simulink model "COMH_Test"  (R2016b)
settings: Solver=VariableStepAuto  StartTime=0.0  StopTime=55  RelTol=1e-3  EnableMultiTasking=on
undefined symbols (not defined in the file or in its folder): CAL_EncoderSampleTime, CAL_fullCircle_DEG, CAL_MeasureNoise, CAL_ProcessNoise, CAL_ROB_ERRVAL, CAL_ROBO_LENG_mm, CAL_thetaGain, COMH, Compass_Handler, CONST_EnableDelay, CONST_ZERO_UINT16, CONST_ZeroDeg, ENU_ROB_NONE, sigbuilder_block
libraries: simulink_need_slupdate x1, ThetaOverFlowFilter x1, movingAverage_1ms_to_5ms x1, simulink x1
settings Model: Creator=oelkawok  LastModifiedBy=oelkawok
settings OptimizationCC: LifeSpan=inf
settings DebuggingCC: SFUnexpectedBacktrackingDiag=warning  SFNoUnconditionalDefaultTransitionDiag=warning  SFExecutionAtInitializationDiag=none
settings GRTTargetCC: TargetLangStandard=C89/C90 (ANSI)  GeneratePreprocessorConditionals=Disable all
settings ConfigComp: CovMetricSettings=dw  CovHtmlReporting=on  CovSaveCumulativeToWorkspaceVar=on  CovSaveSingleToWorkspaceVar=on  CovExternalEMLEnable=off

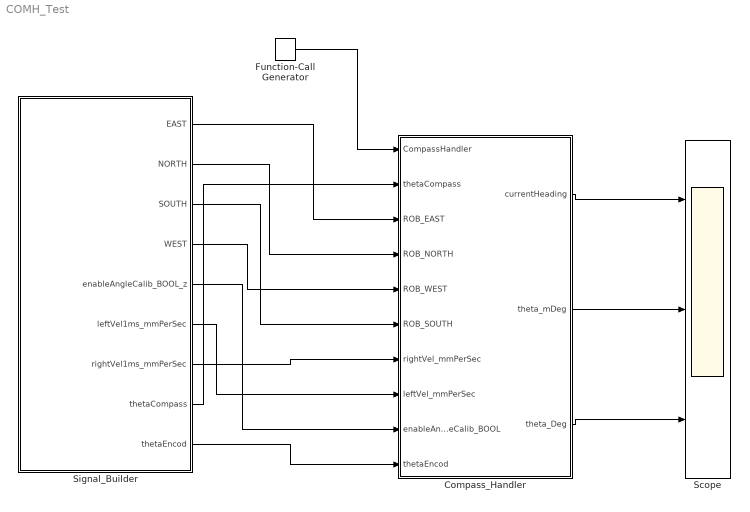
== system COMH_Test ==
  Compass_Handler : Subsystem  AncestorBlock=COMH/Compass_Handler
  Function-Call Generator : simulink/Ports & Subsystems/Function-Call Generator  sample_time=0.005  numberOfIterations=1
  Scope : Scope  NumInputPorts=3
  Signal_Builder : Subsystem  Tag=STV Subsys  LoadFcn=sigbuilder_block('load',[5.4 30 1141.2 522.6 ]);  StartFcn=sigbuilder_block('start');  StopFcn=sigbuilder_block('stop');  ClipboardFcn=sigbuilder_block('clipboard');  mask(Sigbuilder block){tuvar=[0:10]}
      mask help: Simulink:masks:SigbuilderBlock_MD
      mask init:
      | if ~strcmp(get_param(bdroot(gcbh),'SimulationStatus'),'stopped') tuvar = sigbuilder_block('maskInit'); end
      settings: CopyFcn=sigbuilder_block('copy');  DeleteFcn=sigbuilder_block('delete');  ModelCloseFcn=sigbuilder_block('modelClose');  PreSaveFcn=sigbuilder_block('preSave');  PauseFcn=sigbuilder_block('pause');  ContinueFcn=sigbuilder_block('continue');  NameChangeFcn=sigbuilder_block('namechange');  OpenFcn=sigbuilder_block('open',[437.6 199.2 550.4 400 ]);  CloseFcn=sigbuilder_block('close');
      mask Display: plot(0, 0, 100, 100,[2, 2, 32, 32, 2], [68, 8, 8, 68, 68],[32, 2], [38, 38], [32, 19, 2],[53, 60, 44], [32, 17, 17, 2],[16, 16, 31, 31]);txt = getActiveGroup(gcbh);text(2, 100, txt,'verticalAlignment', 'top');
  wires:
  Compass_Handler/1(currentHeading) -> Scope/1
  Signal_Builder/1(EAST) -> Compass_Handler/3(ROB_EAST)
  Signal_Builder/2(NORTH) -> Compass_Handler/4(ROB_NORTH)
  Signal_Builder/4(WEST) -> Compass_Handler/5(ROB_WEST)
  Signal_Builder/3(SOUTH) -> Compass_Handler/6(ROB_SOUTH)
  Signal_Builder/5(enableAngleCalib_BOOL_z) -> Compass_Handler/9(enableAngleCalib_BOOL)
  Signal_Builder/6(leftVel1ms_mmPerSec) -> Compass_Handler/8(leftVel_mmPerSec)
  Signal_Builder/7(rightVel1ms_mmPerSec) -> Compass_Handler/7(rightVel_mmPerSec)
  Signal_Builder/9(thetaEncod) -> Compass_Handler/10(thetaEncod)
  Signal_Builder/8(thetaCompass) -> Compass_Handler/2(thetaCompass)
  Function-Call Generator/1 -> Compass_Handler/1(CompassHandler)
  Compass_Handler/3(theta_Deg) -> Scope/3
  Compass_Handler/2(theta_mDeg) -> Scope/2

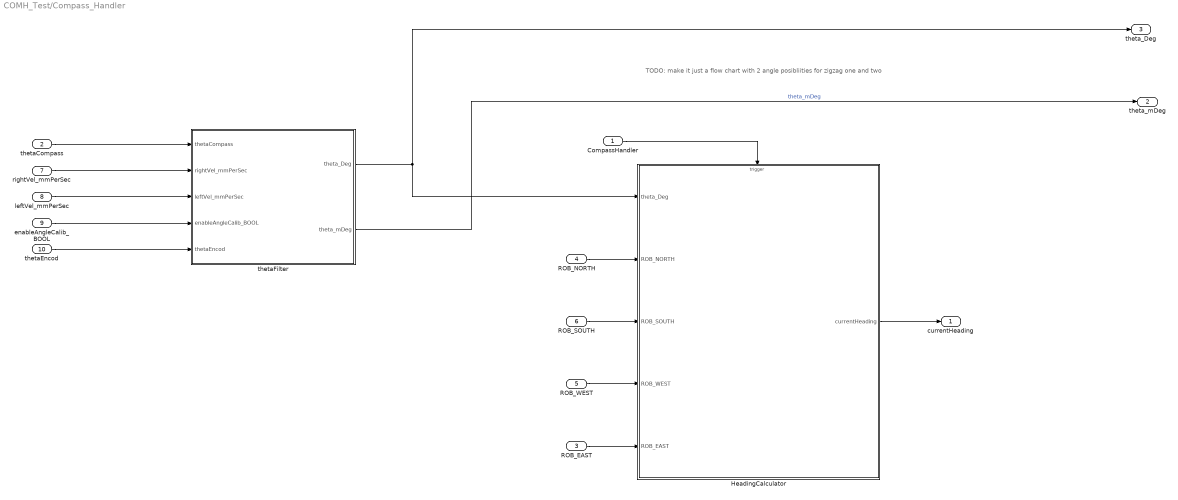
== system COMH_Test/Compass_Handler ==
  note: TODO: make it just a flow chart with 2 angle posibliities for zigzag one and two
  CompassHandler : Inport  PortDimensions=1
  thetaCompass : Inport  Port=2
  ROB_EAST : Inport  Port=3  PortDimensions=1
  ROB_NORTH : Inport  Port=4  PortDimensions=1
  ROB_WEST : Inport  Port=5  PortDimensions=1
  ROB_SOUTH : Inport  Port=6  PortDimensions=1
  rightVel_mmPerSec : Inport  Port=7  PortDimensions=1
  leftVel_mmPerSec : Inport  Port=8  PortDimensions=1
  enableAngleCalib_BOOL : Inport  Port=9
  thetaEncod : Inport  Port=10  PortDimensions=1
  HeadingCalculator : Subsystem
  thetaFilter : Subsystem
  currentHeading : Outport
      settings: AttributesFormatString=|
      | Mode: %<OutputWhenDisabled>
      | Init: %<InitialOutput>
  theta_mDeg : Outport  Port=2
      settings: AttributesFormatString=|
      | Mode: %<OutputWhenDisabled>
      | Init: %<InitialOutput>
  theta_Deg : Outport  Port=3
      settings: AttributesFormatString=|
      | Mode: %<OutputWhenDisabled>
      | Init: %<InitialOutput>
  wires:
  thetaFilter/2(theta_mDeg) -> theta_mDeg/1  "theta_mDeg"
  thetaCompass/1 -> thetaFilter/1(thetaCompass)
  rightVel_mmPerSec/1 -> thetaFilter/2(rightVel_mmPerSec)
  leftVel_mmPerSec/1 -> thetaFilter/3(leftVel_mmPerSec)
  enableAngleCalib_BOOL/1 -> thetaFilter/4(enableAngleCalib_BOOL)
  thetaEncod/1 -> thetaFilter/5(thetaEncod)
  ROB_NORTH/1 -> HeadingCalculator/2(ROB_NORTH)
  ROB_SOUTH/1 -> HeadingCalculator/3(ROB_SOUTH)
  ROB_WEST/1 -> HeadingCalculator/4(ROB_WEST)
  ROB_EAST/1 -> HeadingCalculator/5(ROB_EAST)
  HeadingCalculator/1(currentHeading) -> currentHeading/1
  CompassHandler/1 -> HeadingCalculator/Trigger
  thetaFilter/1(theta_Deg) -> theta_Deg/1, HeadingCalculator/1(theta_Deg)

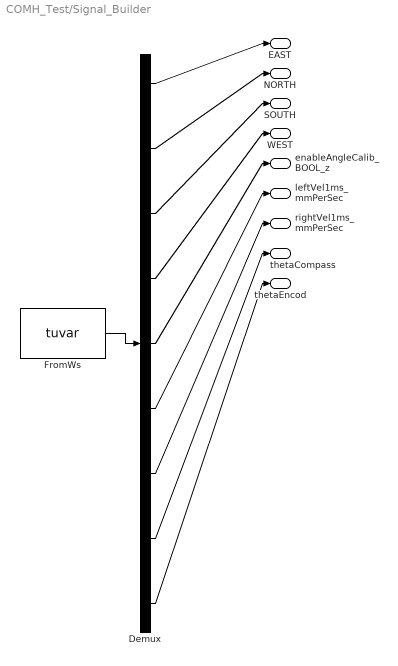
== system COMH_Test/Signal_Builder ==
  Demux : Demux  Tag=STV Demux  Outputs=9
  FromWs : FromWorkspace  Tag=STV FromWs  VariableName=tuvar  SampleTime=0
      SigBuilderData=|
      | common.afterFinalStr = 'Extrapolate'
      | common.sampleTime = 0
      | dataSet.timeRange = [0 55]
      | dataSet.name = 'Group 1'
      | sbobj.Groups.Name = 'Group 1'
      | sbobj.Groups.Signals(1).Name = 'EAST'
      | sbobj.Groups.Signals(1).XData = [0 0.001 0.002 0.003 0.004 0.005 0.006 0.007 0.008 0.009 0.01 0.011 ... (55001 elements, 1x55001)]
      | sbobj.Groups.Signals(1).YData = [0 0 0 0 0 0 0 0 0 0 0 0 ... (55001 elements, 1x55001)]
      | sbobj.Groups.Signals(2).Name = 'NORTH'
      | sbobj.Groups.Signals(2).XData = [0 0.001 0.002 0.003 0.004 0.005 0.006 0.007 0.008 0.009 0.01 0.011 ... (55001 elements, 1x55001)]
      | sbobj.Groups.Signals(2).YData = [0 0 0 0 0 270 270 270 270 270 270 270 ... (55001 elements, 1x55001)]
      | sbobj.Groups.Signals(3).Name = 'SOUTH'
      | sbobj.Groups.Signals(3).XData = [0 0.001 0.002 0.003 0.004 0.005 0.006 0.007 0.008 0.009 0.01 0.011 ... (55001 elements, 1x55001)]
      | sbobj.Groups.Signals(3).YData = [0 0 0 0 0 90 90 90 90 90 90 90 ... (55001 elements, 1x55001)]
      | sbobj.Groups.Signals(4).Name = 'WEST'
      | sbobj.Groups.Signals(4).XData = [0 0.001 0.002 0.003 0.004 0.005 0.006 0.007 0.008 0.009 0.01 0.011 ... (55001 elements, 1x55001)]
      | sbobj.Groups.Signals(4).YData = [0 0 0 0 0 180 180 180 180 180 180 180 ... (55001 elements, 1x55001)]
      | sbobj.Groups.Signals(5).Name = 'enableAngleCalib_BOOL_z'
      | sbobj.Groups.Signals(5).XData = [0 0.001 0.002 0.003 0.004 0.005 0.006 0.007 0.008 0.009 0.01 0.011 ... (55001 elements, 1x55001)]
      | sbobj.Groups.Signals(5).YData = [0 0 0 0 0 0 0 0 0 0 0 0 ... (55001 elements, 1x55001)]
      | sbobj.Groups.Signals(6).Name = 'leftVel1ms_mmPerSec'
      | sbobj.Groups.Signals(6).XData = [0 0.001 0.002 0.003 0.004 0.005 0.006 0.007 0.008 0.009 0.01 0.011 ... (55001 elements, 1x55001)]
      | sbobj.Groups.Signals(6).YData = [0 0 0 0 0 0 -4.02308368683 -13.071685791 -21.6700782776 -29.0321083069 -35.826374054 -37.7429084778 ... (55001 elements, 1x55001)]
      | sbobj.Groups.Signals(7).Name = 'rightVel1ms_mmPerSec'
      | sbobj.Groups.Signals(7).XData = [0 0.001 0.002 0.003 0.004 0.005 0.006 0.007 0.008 0.009 0.01 0.011 ... (55001 elements, 1x55001)]
      | sbobj.Groups.Signals(7).YData = [0 0 0 0 0 0 4.02308368683 13.071685791 21.6700782776 29.0321083069 35.826374054 37.7429084778 ... (55001 elements, 1x55001)]
      | sbobj.Groups.Signals(8).Name = 'thetaCompass'
      | sbobj.Groups.Signals(8).XData = [0 0.001 0.002 0.003 0.004 0.005 0.006 0.007 0.008 0.009 0.01 0.011 ... (55001 elements, 1x55001)]
      | sbobj.Groups.Signals(8).YData = [270 301 300 299 299 298 299 299 299 299 299 299 ... (55001 elements, 1x55001)]
      | sbobj.Groups.Signals(9).Name = 'thetaEncod'
      | sbobj.Groups.Signals(9).XData = [0 0.001 0.002 0.003 0.004 0.005 0.006 0.007 0.008 0.009 0.01 0.011 ... (55001 elements, 1x55001)]
      | sbobj.Groups.Signals(9).YData = [54 108 162 216 270 270 269.999633789 269.998077393 269.994506836 269.988311768 269.978790283 269.966217041 ... (55001 elements, 1x55001)]
      | sbobj.Groups.TimeRange = [0 55]
  EAST : Outport  Tag=STV Outport
  NORTH : Outport  Tag=STV Outport  Port=2
  SOUTH : Outport  Tag=STV Outport  Port=3
  WEST : Outport  Tag=STV Outport  Port=4
  enableAngleCalib_BOOL_z : Outport  Tag=STV Outport  Port=5
  leftVel1ms_mmPerSec : Outport  Tag=STV Outport  Port=6
  rightVel1ms_mmPerSec : Outport  Tag=STV Outport  Port=7
  thetaCompass : Outport  Tag=STV Outport  Port=8
  thetaEncod : Outport  Tag=STV Outport  Port=9
  wires:
  FromWs/1 -> Demux/1
  Demux/1 -> EAST/1
  Demux/2 -> NORTH/1
  Demux/3 -> SOUTH/1
  Demux/4 -> WEST/1
  Demux/5 -> enableAngleCalib_BOOL_z/1
  Demux/6 -> leftVel1ms_mmPerSec/1
  Demux/7 -> rightVel1ms_mmPerSec/1
  Demux/8 -> thetaCompass/1
  Demux/9 -> thetaEncod/1

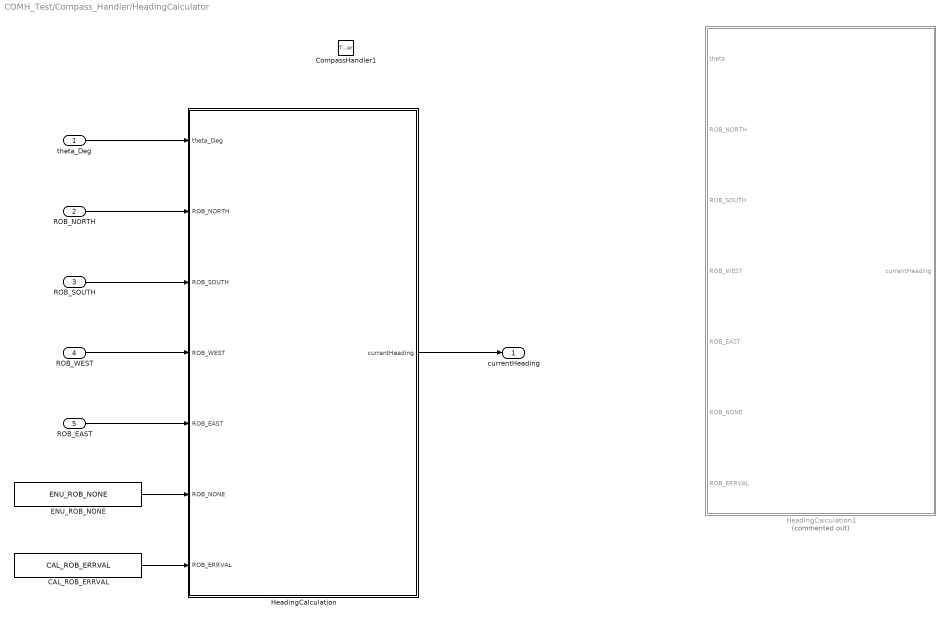
== system COMH_Test/Compass_Handler/HeadingCalculator ==
  theta_Deg : Inport
  ROB_NORTH : Inport  Port=2  PortDimensions=1
  ROB_SOUTH : Inport  Port=3  PortDimensions=1
  ROB_WEST : Inport  Port=4  PortDimensions=1
  ROB_EAST : Inport  Port=5  PortDimensions=1
  CompassHandler1 : TriggerPort  TriggerType=function-call  VariantControl=Variant
      settings: AttributesFormatString=Mode: %<StatesWhenEnabling>
  CAL_ROB_ERRVAL : Constant  Value=CAL_ROB_ERRVAL
  ENU_ROB_NONE : Constant  Value=ENU_ROB_NONE
  HeadingCalculation : Stateflow chart  TreatAsAtomicUnit=on
  HeadingCalculation1 : Stateflow chart  Commented=on  TreatAsAtomicUnit=on
  currentHeading : Outport
      settings: AttributesFormatString=|
      | Mode: %<OutputWhenDisabled>
      | Init: %<InitialOutput>
  wires:
  ENU_ROB_NONE/1 -> HeadingCalculation/6(ROB_NONE)
  CAL_ROB_ERRVAL/1 -> HeadingCalculation/7(ROB_ERRVAL)
  ROB_EAST/1 -> HeadingCalculation/5(ROB_EAST)
  ROB_WEST/1 -> HeadingCalculation/4(ROB_WEST)
  ROB_SOUTH/1 -> HeadingCalculation/3(ROB_SOUTH)
  ROB_NORTH/1 -> HeadingCalculation/2(ROB_NORTH)
  HeadingCalculation/1(currentHeading) -> currentHeading/1
  theta_Deg/1 -> HeadingCalculation/1(theta_Deg)

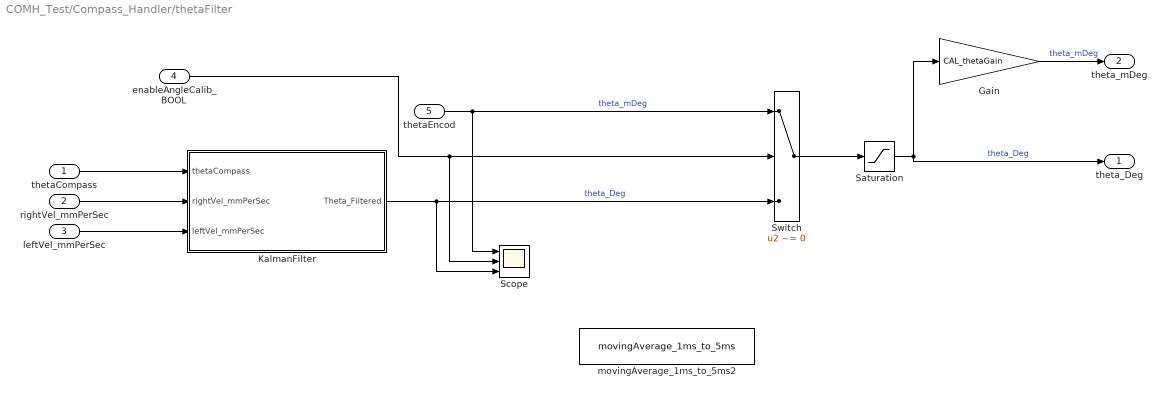
== system COMH_Test/Compass_Handler/thetaFilter ==
  thetaCompass : Inport
  rightVel_mmPerSec : Inport  Port=2  PortDimensions=1
  leftVel_mmPerSec : Inport  Port=3  PortDimensions=1
  enableAngleCalib_BOOL : Inport  Port=4
  thetaEncod : Inport  Port=5  PortDimensions=1
  Gain : Gain  Gain=CAL_thetaGain
  KalmanFilter : Subsystem
  Saturation : Saturate  UpperLimit=CAL_fullCircle_DEG  LowerLimit=CONST_ZERO_UINT16
      settings: AttributesFormatString=|
      | upper = %<UpperLimit>
      | lower = %<LowerLimit>
  Scope : Scope  NumInputPorts=3
  Switch : Switch  Criteria=u2 ~= 0
  movingAverage_1ms_to_5ms2 : movingAverage_1ms_to_5ms/movingAverage_1ms_to_5ms
  theta_Deg : Outport
  theta_mDeg : Outport  Port=2
  wires:
  rightVel_mmPerSec/1 -> KalmanFilter/2(rightVel_mmPerSec)
  leftVel_mmPerSec/1 -> KalmanFilter/3(leftVel_mmPerSec)
  thetaCompass/1 -> KalmanFilter/1(thetaCompass)
  Switch/1 -> Saturation/1
  enableAngleCalib_BOOL/1 -> Scope/2, Switch/2
  Saturation/1 -> theta_Deg/1, Gain/1  "theta_Deg"
  Gain/1 -> theta_mDeg/1  "theta_mDeg"
  thetaEncod/1 -> Switch/1, Scope/1  "theta_mDeg"
  KalmanFilter/1(Theta_Filtered) -> Switch/3, Scope/3  "theta_Deg"

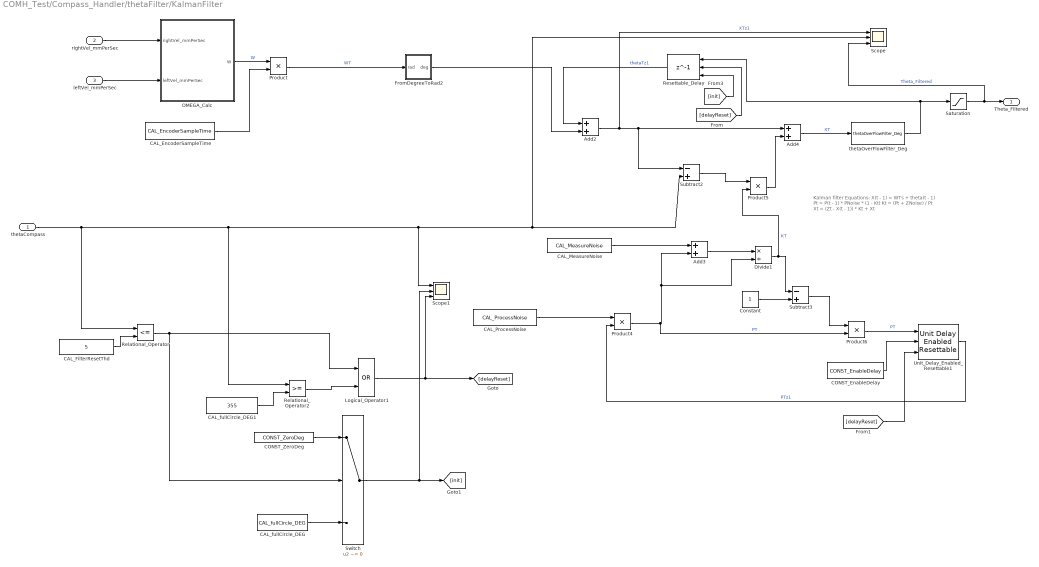
== system COMH_Test/Compass_Handler/thetaFilter/KalmanFilter ==
  note: Kalman filter Equations:
      | X(t - 1) = WTs + theta(t - 1)
      | Pt = P(t - 1) * PNoise * (1 - Kt)
      | Kt = (Pt + ZNoise) / Pt
      | Xt = (Zt - X(t - 1)) * Kt + Xt
  thetaCompass : Inport
  rightVel_mmPerSec : Inport  Port=2
  leftVel_mmPerSec : Inport  Port=3
  Add2 : Sum  OutDataTypeStr=Inherit: Same as first input
  Add3 : Sum
  Add4 : Sum  OutDataTypeStr=single
  CAL_EncoderSampleTime : Constant  Value=CAL_EncoderSampleTime
  CAL_FilterResetThd : Constant  Value=5
  CAL_MeasureNoise : Constant  Value=CAL_MeasureNoise
  CAL_ProcessNoise : Constant  Value=CAL_ProcessNoise
  CAL_fullCircle_DEG : Constant  Value=CAL_fullCircle_DEG
  CAL_fullCircle_DEG1 : Constant  Value=355
  CONST_EnableDelay : Constant  Value=CONST_EnableDelay
  CONST_ZeroDeg : Constant  Value=CONST_ZeroDeg
  Constant : Constant  OutDataTypeStr=single
  Divide1 : Product  Inputs=*/  OutDataTypeStr=Inherit: Inherit via back propagation
  FromDegreeToRad2 : Subsystem
  Logical_Operator1 : Logic  Operator=OR  AllPortsSameDT=off  OutDataTypeStr=boolean
  OMEGA_Calc : Subsystem
  Product : Product
  Product4 : Product  OutDataTypeStr=Inherit: Inherit via back propagation
  Product5 : Product  OutDataTypeStr=single
  Product6 : Product  OutDataTypeStr=Inherit: Inherit via back propagation
  Relational_Operator : RelationalOperator  Operator=<=  OutDataTypeStr=boolean  RndMeth=Nearest
  Relational_Operator2 : RelationalOperator  OutDataTypeStr=boolean  RndMeth=Nearest
  Resettable_Delay : Delay  DelayLength=1  InitialConditionSource=Input port  ExternalReset=Rising
      settings: AttributesFormatString=Init: %<InitialCondition>  InputPortMap=u0,r5,p4
  Saturation : Saturate  UpperLimit=360  LowerLimit=0
      settings: AttributesFormatString=|
      | upper = %<UpperLimit>
      | lower = %<LowerLimit>
  Scope : Scope  NumInputPorts=3
  Scope1 : Scope  NumInputPorts=3
  Subtract2 : Sum  Inputs=-+
  Subtract3 : Sum  Inputs=-+  OutDataTypeStr=Inherit: Inherit via back propagation
  Switch : Switch  Criteria=u2 ~= 0
  Unit_Delay_Enabled_Resettable1 : simulink_need_slupdate/Unit Delay Enabled Resettable  vinit=1  tsamp=-1
  thetaOverFlowFilter_Deg : ThetaOverFlowFilter/thetaOverFlowFilter_Deg
  Theta_Filtered : Outport
  wires:
  leftVel_mmPerSec/1 -> OMEGA_Calc/2(leftVel_mmPerSec)
  rightVel_mmPerSec/1 -> OMEGA_Calc/1(rightVel_mmPerSec)
  CAL_EncoderSampleTime/1 -> Product/2
  OMEGA_Calc/1(W) -> Product/1  "W"
  thetaCompass/1 -> Relational_Operator/1, Relational_Operator2/1, Scope1/1, Scope/2, Subtract2/2
  Product/1 -> FromDegreeToRad2/1(rad)  "WT"
  Resettable_Delay/1 -> Add2/1  "thetaTz1"
  CAL_ProcessNoise/1 -> Product4/1
  Unit_Delay_Enabled_Resettable1/1 -> Product4/2  "PTz1"
  Product4/1 -> Product6/2, Divide1/2, Add3/2  "PT"
  CAL_MeasureNoise/1 -> Add3/1
  Add3/1 -> Divide1/1
  Divide1/1 -> Subtract3/1, Product5/2  "KT"
  Add2/1 -> Scope/1, Subtract2/1, Add4/1  "XTz1"
  Subtract2/1 -> Product5/1
  Constant/1 -> Subtract3/2
  Subtract3/1 -> Product6/1
  Product6/1 -> Unit_Delay_Enabled_Resettable1/1  "PT"
  Product5/1 -> Add4/2
  Add4/1 -> thetaOverFlowFilter_Deg/1  "XT"
  CAL_FilterResetThd/1 -> Relational_Operator/2
  [delayReset] -> Resettable_Delay/2
  CONST_EnableDelay/1 -> Unit_Delay_Enabled_Resettable1/2
  [delayReset] -> Unit_Delay_Enabled_Resettable1/3
  thetaOverFlowFilter_Deg/1 -> Resettable_Delay/1, Saturation/1
  Saturation/1 -> Scope/3, Theta_Filtered/1  "Theta_Filtered"
  CONST_ZeroDeg/1 -> Switch/1
  CAL_fullCircle_DEG/1 -> Switch/3
  [init] -> Resettable_Delay/3
  FromDegreeToRad2/1(deg) -> Add2/2
  Logical_Operator1/1 -> [delayReset], Scope1/3
  Switch/1 -> [init], Scope1/2
  Relational_Operator/1 -> Switch/2, Logical_Operator1/1
  Relational_Operator2/1 -> Logical_Operator1/2
  CAL_fullCircle_DEG1/1 -> Relational_Operator2/2

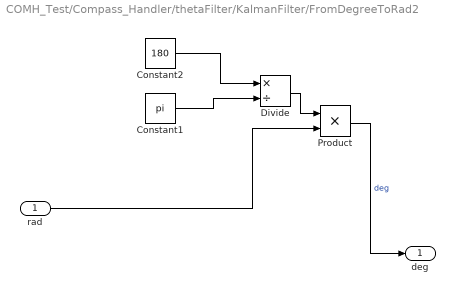
== system COMH_Test/Compass_Handler/thetaFilter/KalmanFilter/FromDegreeToRad2 ==
  rad : Inport
  Constant1 : Constant  Value=pi
  Constant2 : Constant  Value=180
  Divide : Product  Inputs=*/
  Product : Product
  deg : Outport
  wires:
  Divide/1 -> Product/1
  rad/1 -> Product/2
  Product/1 -> deg/1  "deg"
  Constant2/1 -> Divide/1
  Constant1/1 -> Divide/2

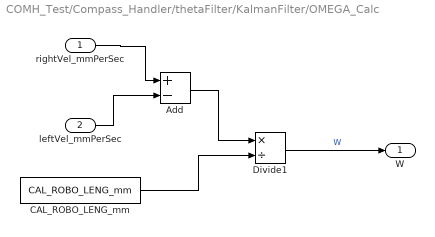
== system COMH_Test/Compass_Handler/thetaFilter/KalmanFilter/OMEGA_Calc ==
  rightVel_mmPerSec : Inport
  leftVel_mmPerSec : Inport  Port=2
  Add : Sum  Inputs=+-
  CAL_ROBO_LENG_mm : Constant  Value=CAL_ROBO_LENG_mm
  Divide1 : Product  Inputs=*/  OutDataTypeStr=single
  W : Outport
  wires:
  leftVel_mmPerSec/1 -> Add/2
  rightVel_mmPerSec/1 -> Add/1
  CAL_ROBO_LENG_mm/1 -> Divide1/2
  Divide1/1 -> W/1  "W"
  Add/1 -> Divide1/1

== stateflow chart COMH_Test/Compass_Handler/HeadingCalculator/HeadingCalculation1 ==
  settings: description=Chart for calculation of heading. Could be used as state but not used
  state CalcHeadingEastZero
    (default) -> (junction 2)
    (junction 2) -> (junction 3) [order 1] : [(theta_OUT <= ROB_NORTH + ROB_ERRVAL) && (theta_OUT >= ROB_NORTH - ROB_ERRVAL)]//NORTH
    (junction 2) -> (junction 4) [order 2]
    (junction 3) -> (junction 17) : {currentHeading = ROB_NORTH;}
    (junction 4) -> (junction 5) [order 1] : [(theta_OUT <= ROB_SOUTH + ROB_ERRVAL) && (theta_OUT >= ROB_SOUTH - ROB_ERRVAL)]//SOUTH
    (junction 4) -> (junction 6) [order 2]
    (junction 5) -> (junction 16) : {currentHeading = ROB_SOUTH;}
    (junction 6) -> (junction 7) [order 1] : [(theta_OUT <= ROB_EAST + ROB_ERRVAL) || (theta_OUT >= CAL_fullCircle_DEG - ROB_ERRVAL)]//EAST
    (junction 6) -> (junction 8) [order 2]
    (junction 7) -> (junction 15) : {currentHeading = ROB_EAST;}
    (junction 8) -> (junction 9) [order 1] : [(theta_OUT <= ROB_WEST + ROB_ERRVAL) && (theta_OUT >= ROB_WEST - ROB_ERRVAL)]//WEST
    (junction 8) -> (junction 12) [order 2] : {currentHeading = ROB_NONE;}
    (junction 9) -> (junction 14) : {currentHeading = ROB_WEST;}
    (junction 14) -> (junction 12)
    (junction 15) -> (junction 14)
    (junction 16) -> (junction 15)
    (junction 17) -> (junction 16)
    (junction 12) -> (junction 18)
  state initializeDirection
    entry:
    offset = theta;
  state Calc
    entry:
    theta_OUT = theta;
    //remove for now - offset
  state CalcHeadingSouthZero
    (default) -> (junction 68)
    (junction 68) -> (junction 69) [order 1] : [(theta_OUT <= ROB_NORTH + ROB_ERRVAL) && (theta_OUT >= ROB_NORTH - ROB_ERRVAL)]//NORTH
    (junction 68) -> (junction 70) [order 2]
    (junction 69) -> (junction 80) : {currentHeading = ROB_NORTH;}
    (junction 70) -> (junction 71) [order 1] : [(theta_OUT <= ROB_SOUTH + ROB_ERRVAL) || (theta_OUT >= CAL_fullCircle_DEG - ROB_ERRVAL)]//SOUTH
    (junction 70) -> (junction 72) [order 2]
    (junction 71) -> (junction 79) : {currentHeading = ROB_SOUTH;}
    (junction 72) -> (junction 73) [order 1] : [(theta_OUT <= ROB_EAST + ROB_ERRVAL) && (theta_OUT >= ROB_EAST - ROB_ERRVAL)]//EAST
    (junction 72) -> (junction 74) [order 2]
    (junction 73) -> (junction 78) : {currentHeading = ROB_EAST;}
    (junction 74) -> (junction 75) [order 1] : [(theta_OUT <= ROB_WEST + ROB_ERRVAL) && (theta_OUT >= ROB_WEST - ROB_ERRVAL)]//WEST
    (junction 74) -> (junction 76) [order 2] : {currentHeading = ROB_NONE;}
    (junction 75) -> (junction 77) : {currentHeading = ROB_WEST;}
    (junction 77) -> (junction 76)
    (junction 78) -> (junction 77)
    (junction 79) -> (junction 78)
    (junction 80) -> (junction 79)
    (junction 76) -> (junction 81)
  CalcHeadingEastZero -> (junction 64) : /theta_OUT = theta;
  (junction 64) -> CalcHeadingEastZero [order 1] : [ROB_EAST == 0]
  Calc -> (junction 64) [order 2] : [hasChanged(theta)]
  CalcHeadingSouthZero -> (junction 64) : /theta_OUT = theta;
  (junction 64) -> CalcHeadingSouthZero [order 2] : [ROB_SOUTH == 0]
  Calc -> (junction 64) [order 3] : [theta_OUT < 0]
      | /
      | theta_OUT := theta_OUT + CAL_fullCircle_DEG;
  (junction 57) -> (junction 64) : /theta_OUT = ROB_ERRVAL;
  (junction 64) -> Calc [order 3]
  (default) -> initializeDirection
  initializeDirection -> Calc
  Calc -> (junction 57) [order 1] : [theta_OUT < ROB_ERRVAL]
  data: theta input; ROB_NORTH input; ROB_SOUTH input; ROB_WEST input; ROB_EAST input; ROB_NONE input; ROB_ERRVAL input; theta_OUT local int16; currentHeading output uint16; offset local int16; CAL_fullCircle_DEG constant uint16 =CAL_fullCircle_DEG

== stateflow chart COMH_Test/Compass_Handler/HeadingCalculator/HeadingCalculation ==
  settings: description=Chart for calculation of heading. Could be used as state but not used
  (default) -> (junction 109)
  (junction 109) -> (junction 110) [order 1] : [(theta_Deg <= ROB_NORTH + ROB_ERRVAL) && (theta_Deg >= ROB_NORTH - ROB_ERRVAL)]//NORTH
  (junction 109) -> (junction 103) [order 2]
  (junction 110) -> (junction 116) : {currentHeading = ROB_NORTH;}
  (junction 103) -> (junction 106) [order 1] : [(theta_Deg <= ROB_SOUTH + ROB_ERRVAL) && (theta_Deg >= ROB_SOUTH - ROB_ERRVAL)]//SOUTH
  (junction 103) -> (junction 104) [order 2]
  (junction 106) -> (junction 119) : {currentHeading = ROB_SOUTH;}
  (junction 104) -> (junction 107) [order 1] : [(theta_Deg <= ROB_EAST + ROB_ERRVAL) || (theta_Deg >= CAL_fullCircle_DEG - ROB_ERRVAL)]//EAST
  (junction 104) -> (junction 105) [order 2]
  (junction 107) -> (junction 115) : {currentHeading = ROB_EAST;}
  (junction 105) -> (junction 108) [order 1] : [(theta_Deg <= ROB_WEST + ROB_ERRVAL) && (theta_Deg >= ROB_WEST - ROB_ERRVAL)]//WEST
  (junction 105) -> (junction 113) [order 2] : {currentHeading = ROB_NONE;}
  (junction 108) -> (junction 114) : {currentHeading = ROB_WEST;}
  (junction 114) -> (junction 113)
  (junction 115) -> (junction 114)
  (junction 119) -> (junction 115)
  (junction 116) -> (junction 119)
  (junction 113) -> (junction 117)
  data: theta_Deg input; ROB_NORTH input; ROB_SOUTH input; ROB_WEST input; ROB_EAST input; ROB_NONE input; ROB_ERRVAL input; currentHeading output uint16; CAL_fullCircle_DEG constant uint16 =CAL_fullCircle_DEG
